simulink model "model1"  (R2024a)
settings: Solver=ode23t  StartTime=0.0  StopTime=TimeMax  MaxStep=0.1  RelTol=1e-3
model workspace (MAT data in the model file):
  con = [27 27 27 27 27 27 27 28 28 27 27 28 ... (60 elements, 1x60)]
  novar = 30
  varray = [28 29 27 30 26 28 29 27 25 30 28 29 ... (60 elements, 1x60)]
undefined symbols (not defined in the file): AirDensity, CD, CRR, DistancetoGlide, finalatt, FrontArea, FrontAxle, FrontGear, Gravitation, MassWheel, NewData, RadiusWheel, RearAxle, RearGear, SlipAngle, StateData, TrackData, VehicleMass
libraries: fl_lib x18, nesl_utility x14, sdl_lib x7, ee_lib x2, batteryecm_lib x1
(part 2 of 2)

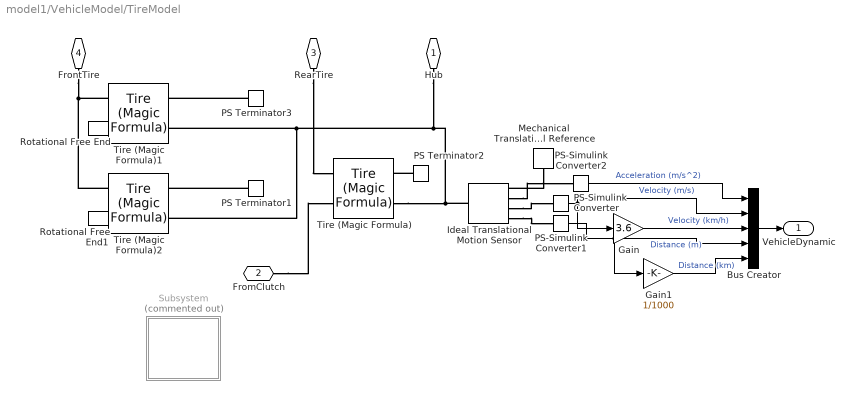
== system model1/VehicleModel/TireModel ==
  Bus Creator : BusCreator  Inputs=5
  Gain : Gain  Gain=3.6
  Gain1 : Gain  Gain=1/1000
  Ideal Translational Motion Sensor : fl_lib/Mechanical/Mechanical Sensors/Ideal Translational Motion Sensor  reference=foundation.enum.MeasurementReference.difference  acceleration_port=true  velocity_port=true  position_port=true  offset=0 m
      settings: InternalSimscapePortConfiguration="{\"Bottom\":[],\"Left\":[{\"id\":\"R\",\"label\":\"R\",\"type\":\"foundation.mechanical.translational.translational\"}],\"Right\":[{\"id\":\"C\",\"label\":\"C\",\"type\":\"foundation.mechanical.translational.translational\"},{\"id\":\"A\",\"label\":\"A\",\"type\":\"output\"},{\"id\":\"V\",\"label\":\"V\",\"type\":\"output\"},{\"id\":\"P\",\"label\":\"P\",\"type\":\"output\"}],\"Top\":[]}"
  Mechanical Translational Reference : fl_lib/Mechanical/Translational Elements/Mechanical Translational Reference
  PS Terminator1 : fl_lib/Physical Signals/Sinks/PS Terminator
  PS Terminator2 : fl_lib/Physical Signals/Sinks/PS Terminator
  PS Terminator3 : fl_lib/Physical Signals/Sinks/PS Terminator
  PS-Simulink Converter : nesl_utility/PS-Simulink Converter  PhysicalDomain=network_engine_domain  SubClassName=ps_output  LeftPortType=input  RightPortType=output  PseudoPeriodic=off  Frequencies=[]  VectorFormat=1-D array  Unit=m/s  AffineConversion=off
  PS-Simulink Converter1 : nesl_utility/PS-Simulink Converter  PhysicalDomain=network_engine_domain  SubClassName=ps_output  LeftPortType=input  RightPortType=output  PseudoPeriodic=off  Frequencies=[]  VectorFormat=1-D array  Unit=m  AffineConversion=off
  PS-Simulink Converter2 : nesl_utility/PS-Simulink Converter  PhysicalDomain=network_engine_domain  SubClassName=ps_output  LeftPortType=input  RightPortType=output  PseudoPeriodic=off  Frequencies=[]  VectorFormat=1-D array  Unit=m/s^2  AffineConversion=off
  Rotational Free End : fl_lib/Mechanical/Rotational Elements/Rotational Free End  w_specify=off  w_priority=None  w=0 rad/s  w_nominal_specify=off  w_nominal_value=1  w_nominal_unit=rad/s
  Rotational Free End1 : fl_lib/Mechanical/Rotational Elements/Rotational Free End  w_specify=off  w_priority=None  w=0 rad/s  w_nominal_specify=off  w_nominal_value=1  w_nominal_unit=rad/s
  Subsystem : Subsystem  Commented=on
  Tire (Magic Formula) : sdl_lib/Tires & Vehicles/Tire (Magic Formula)  parameterization=sdl.enum.magic_tire_model.peak  F_z1=3000 N  F_x1=3500 N  kappa1=10  B_m=10  C_m=1.9  D_m=1  E_m=0.97  fz0=4000 N  p_Cx=1.685  p_Dx=[1.21, -.037]  p_Ex=[.344, .095, -.02, 0]  p_Kx=[21.51, -.163, .245]  p_Hx=[-.002, .002]  p_Vx=[0, 0]  rolling_radius_model=sdl.enum.RollingRadiusParameterization.Constant  r_e=RadiusWheel m  r_0=0.3 m  breff=8.39  dreff=0.26  freff=0.074  q_re0=0.99  q_v1=0.008  longvl=17 m/s  cz=5e5 N/m  model_resistance=true  resistance_model=sdl.enum.rollingResistanceParameterization.constant  coeff=CRR  p_tire=250e3 Pa  alpha=-0.003  beta=0.97  coeff_a=84e-4  coeff_b=6.2e-4 s/m  coeff_c=1.6e-4 s^2/m^2  p_tire0=240e3 Pa  fz0_resistance=4000 N  vH0=16 m/s  q_Sy=[.0082, 0, .0014, .001, 0, 0, 1.08, -.5]  v_thr=0.001 m/s  enable_scaling_coefficients=false  lfzO=1  lcx=1  lmux=1  lex=1  lkx=1  lhx=1  lvx=1  lmy=1  model_compliance=sdl.enum.compliance.off  stiffness=1e6 N/m  damping=1000 N*s/m  model_inertia=sdl.enum.model_inertia.on  inertia=MassWheel*RadiusWheel^2 kg*m^2  initial_velocity=0 rad/s  vxlow=1 m/s  v_tr_thr=0.1 m/s  kpumin=-1.5  kpumax=1.5
  Tire (Magic Formula)1 : sdl_lib/Tires & Vehicles/Tire (Magic Formula)  parameterization=sdl.enum.magic_tire_model.peak  F_z1=3000 N  F_x1=3500 N  kappa1=10  B_m=10  C_m=1.9  D_m=1  E_m=0.97  fz0=4000 N  p_Cx=1.685  p_Dx=[1.21, -.037]  p_Ex=[.344, .095, -.02, 0]  p_Kx=[21.51, -.163, .245]  p_Hx=[-.002, .002]  p_Vx=[0, 0]  rolling_radius_model=sdl.enum.RollingRadiusParameterization.Constant  r_e=RadiusWheel m  r_0=0.3 m  breff=8.39  dreff=0.26  freff=0.074  q_re0=0.99  q_v1=0.008  longvl=17 m/s  cz=5e5 N/m  model_resistance=true  resistance_model=sdl.enum.rollingResistanceParameterization.constant  coeff=CRR  p_tire=250e3 Pa  alpha=-0.003  beta=0.97  coeff_a=84e-4  coeff_b=6.2e-4 s/m  coeff_c=1.6e-4 s^2/m^2  p_tire0=240e3 Pa  fz0_resistance=4000 N  vH0=16 m/s  q_Sy=[.0082, 0, .0014, .001, 0, 0, 1.08, -.5]  v_thr=0.001 m/s  enable_scaling_coefficients=false  lfzO=1  lcx=1  lmux=1  lex=1  lkx=1  lhx=1  lvx=1  lmy=1  model_compliance=sdl.enum.compliance.off  stiffness=1e6 N/m  damping=1000 N*s/m  model_inertia=sdl.enum.model_inertia.on  inertia=MassWheel*RadiusWheel^2 kg*m^2  initial_velocity=0 rad/s  vxlow=1 m/s  v_tr_thr=0.1 m/s  kpumin=-1.5  kpumax=1.5
  Tire (Magic Formula)2 : sdl_lib/Tires & Vehicles/Tire (Magic Formula)  parameterization=sdl.enum.magic_tire_model.peak  F_z1=3000 N  F_x1=3500 N  kappa1=10  B_m=10  C_m=1.9  D_m=1  E_m=0.97  fz0=4000 N  p_Cx=1.685  p_Dx=[1.21, -.037]  p_Ex=[.344, .095, -.02, 0]  p_Kx=[21.51, -.163, .245]  p_Hx=[-.002, .002]  p_Vx=[0, 0]  rolling_radius_model=sdl.enum.RollingRadiusParameterization.Constant  r_e=RadiusWheel m  r_0=0.3 m  breff=8.39  dreff=0.26  freff=0.074  q_re0=0.99  q_v1=0.008  longvl=17 m/s  cz=5e5 N/m  model_resistance=true  resistance_model=sdl.enum.rollingResistanceParameterization.constant  coeff=CRR  p_tire=250e3 Pa  alpha=-0.003  beta=0.97  coeff_a=84e-4  coeff_b=6.2e-4 s/m  coeff_c=1.6e-4 s^2/m^2  p_tire0=240e3 Pa  fz0_resistance=4000 N  vH0=16 m/s  q_Sy=[.0082, 0, .0014, .001, 0, 0, 1.08, -.5]  v_thr=0.001 m/s  enable_scaling_coefficients=false  lfzO=1  lcx=1  lmux=1  lex=1  lkx=1  lhx=1  lvx=1  lmy=1  model_compliance=sdl.enum.compliance.off  stiffness=1e6 N/m  damping=1000 N*s/m  model_inertia=sdl.enum.model_inertia.on  inertia=MassWheel*RadiusWheel^2 kg*m^2  initial_velocity=0 rad/s  vxlow=1 m/s  v_tr_thr=0.1 m/s  kpumin=-1.5  kpumax=1.5
  Hub : PMIOPort  Side=Left
  FromClutch : PMIOPort  Port=2  Side=Left
  RearTire : PMIOPort  Port=3  Side=Left
  FrontTire : PMIOPort  Port=4  Side=Left
  VehicleDynamic : Outport
  wires:
  PS-Simulink Converter1/1 -> Gain1/1, Bus Creator/4  "Distance (m)"
  PS-Simulink Converter/1 -> Bus Creator/2, Gain/1  "Velocity (m/s)"
  Gain/1 -> Bus Creator/3  "Velocity (km/h)"
  Bus Creator/1 -> VehicleDynamic/1
  Gain1/1 -> Bus Creator/5  "Distance (km)"
  PS-Simulink Converter2/1 -> Bus Creator/1  "Acceleration (m/s^2)"
  connections:
  PS Terminator3/LConn1 -- Tire (Magic Formula)1/RConn1
  FrontTire/RConn1 -- Tire (Magic Formula)1/LConn1 -- Tire (Magic Formula)2/LConn1
  Tire (Magic Formula)/RConn2 -- Ideal Translational Motion Sensor/LConn1 -- Hub/RConn1 -- Tire (Magic Formula)1/RConn2 -- Tire (Magic Formula)2/RConn2
  Tire (Magic Formula)1/LConn2 -- Rotational Free End/LConn1
  Tire (Magic Formula)2/LConn2 -- Rotational Free End1/LConn1
  PS Terminator1/LConn1 -- Tire (Magic Formula)2/RConn1
  RearTire/RConn1 -- Tire (Magic Formula)/LConn1
  PS Terminator2/LConn1 -- Tire (Magic Formula)/RConn1
  FromClutch/RConn1 -- Tire (Magic Formula)/LConn2
  Mechanical Translational Reference/LConn1 -- Ideal Translational Motion Sensor/RConn1
  Ideal Translational Motion Sensor/RConn4 -- PS-Simulink Converter1/LConn1
  Ideal Translational Motion Sensor/RConn3 -- PS-Simulink Converter/LConn1
  Ideal Translational Motion Sensor/RConn2 -- PS-Simulink Converter2/LConn1

== system model1/VehicleModel/TireModel/Subsystem ==
  PS-Simulink Converter2 : nesl_utility/PS-Simulink Converter  PhysicalDomain=network_engine_domain  SubClassName=ps_output  LeftPortType=input  RightPortType=output  PseudoPeriodic=off  Frequencies=[]  VectorFormat=inherit  Unit=inherit  AffineConversion=off
  Road Profile : sdl_lib/Tires & Vehicles/Road Profile  x_f=FrontAxle mm  x_r=RearAxle mm  x_height_vector=TrackData{:,1} m  height_vector=TrackData{:,6} m  friction_output=sdl.enum.tire_friction_model.none  x_friction_vector=[-10, 2, 2.1, 6, 6.1, 10] m  MF_M_matrix=[10, 2, 1, 1; 10, 2, 1, 1; 8, 3, 1, 1; 8, 3, 1, 1; 9, 4, 1, 1; 9, 4, 1, 1]  MR_M_matrix=[10, 2, 1, 1; 10, 2, 1, 1; 8, 3, 1, 1; 8, 3, 1, 1; 9, 4, 1, 1; 9, 4, 1, 1]  MF_F_matrix=[.9, .7; .9, .7; .7, .5; .7, .5; .8, .6; .8, .6]  MR_F_matrix=[.9, .7; .9, .7; .7, .5; .7, .5; .8, .6; .8, .6]  x_specify=off  x_priority=High  x=0 m  x_nominal_specify=off  x_nominal_value=1  x_nominal_unit=m
      settings: InternalSimscapePortConfiguration="{\"Bottom\":[],\"Left\":[],\"Right\":[{\"id\":\"H\",\"label\":\"H\",\"type\":\"foundation.mechanical.translational.translational\"},{\"id\":\"beta\",\"label\":\"beta\",\"type\":\"output\"}],\"Top\":[]}"
  Scope : Scope
  Conn1 : PMIOPort  Side=Right
  wires:
  PS-Simulink Converter2/1 -> Scope/1
  connections:
  PS-Simulink Converter2/LConn1 -- Road Profile/RConn2
  Road Profile/RConn1 -- Conn1/RConn1

== matlab function model1/TurningModel/MATLAB Function1 ==
  data: s input; position output; s_track input
function position = fcn(s, s_track)

if s <= s_track
    position = ceil(s);
else
    position = ceil(s - (ceil(s/s_track) - 1)*s_track);
end

== matlab function model1/TurningModel/MATLAB Function ==
  data: kappa input; F_turn output; v input; m input; sf input; sr input; l input; alpha_f input; alpha_r input
function F_turn = calculate_turn_resistance(kappa, v, m,sf,sr,l,alpha_f,alpha_r)
% Calculate turn resistance force
% Inputs:
%   kappa - curvature (rad/m)
%   v - velocity (m/s)
%   m - mass (kg)
%   sf - CoM to front axle (m)
%   sr - CoM to rear axle (m)
%   l - wheelbase (m)
%   alpha_f - front slip angle (rad)
%   alpha_r - rear slip angle (rad)

% Avoid division by zero

if abs(kappa) < 1e-6
    R_turn = 1e6;  % Very large radius for straight line
else
    R_turn = 1 / kappa;
end

% Calculate turn resistance
mv2 = m * v^2;
slip_term = sf * alpha_f + sr * alpha_r;
F_turn = (mv2 / (R_turn * l)) * slip_term;

% Ensure non-negative force
F_turn = abs(F_turn);
end

== matlab function model1/StateProcessingMayanGacor/MATLAB Function ==
  data: speed input; output output; previousOutput input; accelerationCount output; previousCount input
function [output, accelerationCount] = speedController(speed, previousOutput, previousCount)
% Fungsi kontrol kecepatan dengan hysteresis untuk Simulink
% Input:
%   speed - kecepatan saat ini (kmph)
%   previousOutput - output sebelumnya (0 atau 1)
%   previousCount - jumlah counter sebelumnya
% Output:
%   output - 1 (gas) atau 0 (lepas)
%   accelerationCount - jumlah total percepatan (transisi 0→1)

% Threshold
THRESHOLD_LOW = 24;   % Threshold bawah (set)
THRESHOLD_HIGH = 28;  % Threshold atas (reset)

% Logika hysteresis
if speed <= THRESHOLD_LOW
    output = 1;  % Gas
elseif speed >= THRESHOLD_HIGH
    output = 0;  % Lepas
else
    % Zona tengah (24-28): pertahankan status sebelumnya
    output = previousOutput;
end

% Counter ketika terjadi transisi 0 ke 1
if previousOutput == 0 && output == 1
    accelerationCount = previousCount + 1;
else
    accelerationCount = previousCount;
end

end

== matlab function model1/Inclination Model/MATLAB Function1 ==
  data: s input; position output; s_track input
function position = fcn(s, s_track)

if s <= s_track
    position = ceil(s);
else
    position = ceil(s - (ceil(s/s_track) - 1)*s_track);
end

== matlab function model1/DriverModel/MATLAB Function ==
  data: no_var input; v_array input; control output; v input; state_prev input; n_prev input; state output; n output
function [control,state,n] = fcn(no_var,v_array,v,state_prev,n_prev)

if (n_prev+1) < v_array(no_var*2)
    if state_prev == 0
        if v < v_array(n_prev+1)
            state = 0;
            control = 1;
            n = n_prev;
        else
            state = 1;
            control = 0;
            n = n_prev;
        end
    else
        if v <= v_array(n_prev+1+no_var)
            state = 0;
            control = 1;
            n = n_prev+1;
        else
            state = 1;
            control = 0;
            n = n_prev;
        end
    end
else
    if state_prev == 0
        if v < v_array(n_prev+1)
            state = 0;
            control = 1;
            n = n_prev;
        else
            state = 1;
            control = 0;
            n = n_prev;
        end
    else
        state = 1;
        control = 0;
        n = n_prev;
    end
end
